simulink model "collection_of_goodies"  (Simulink 5.0)
settings: Solver=ode45  StartTime=0.0  StopTime=10.0  RelTol=1e-3
values from neighbouring files (symbols this model uses):
  c = 4.4*tp/(pi*ts)    [PD_sketch_design.m]
  I = [Ixx,Ixy,Ixz;Iyx,Iyy,Iyz;Izx,Izy,Izz]    [starshotmath.m]
  q0 = [qmatlab(2:4),qmatlab(1)]'    [starshot_DC_KD_setup.m]    (also in starshot_DC_setup.m; temp.m)
  s = tf('s')    [starshot_DC_setup.m]
undefined symbols (not defined in the file or in its folder): a1_T_CMG, a2_T_CMG, a3_T_CMG, AccLim, b1_T_CMG, b2_T_CMG, b3_T_CMG, CFthreshoff, CFthreshon, filt1d, filt1n, filt2d, filt2n, filts1n, filts2d, filts2n, fine, h, h_cos_cmg, h_init, h_sin_cmg, hdmax, hmax, I34, Id, Igm1d, Igm1n, IgmAAFd, invI, invId, Is, Isat, IsatSp, k1_obs, k2_obs, Kt, Kts, lam, Lgm, ls, lt, M34, muE, Ngear, P0, pfd, pfn, q_init, r0, rc_ampl, rc_harm, rc_phase, Rgm, Smin, SmotDrag, spin_init, TachAAFd, TAU_ACS, tr_ampl, tr_harm ... (+8)
libraries: simulink x27, mblibv1 x3, dspinverses x1
(part 1 of 2)
settings Model: LastModifiedBy=E150327

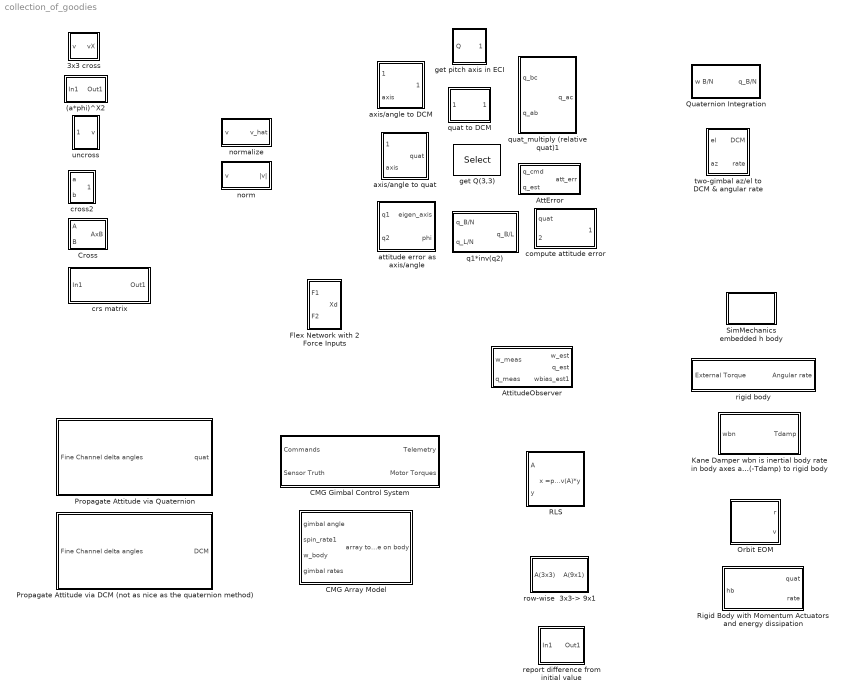
== system collection_of_goodies ==
  " two-gimbal az/el to DCM & angular rate" : Subsystem
  (a*phi)^X2 : Subsystem
      mask Display: disp('3x3 cross')
  3x3 cross : Subsystem
  AttError : Subsystem
  AttitudeObserver : Subsystem
  CMG Array Model : Subsystem
  CMG Gimbal Control System : Subsystem
  Cross : Subsystem
  Flex Network with 2 Force Inputs : Subsystem
  Kane Damper wbn is inertial body rate in body axes apply (-Tdamp) to rigid body : Subsystem
  Orbit EOM : Subsystem
  Propagate Attitude via DCM (not as nice as the quaternion method) : Subsystem
  Propagate Attitude via Quaternion : Subsystem
  Quaternion Integration : Subsystem
  RLS : Subsystem
  Rigid Body with Momentum Actuators and energy dissipation : Subsystem
  SimMechanics embedded h body : Subsystem
  attitude error as axis/angle : Subsystem
  axis/angle to DCM : Subsystem
  axis/angle to quat : Subsystem
  compute attitude error : Subsystem
  cross2 : Subsystem
  crs matrix : Subsystem
  get Q(3,3) : Selector  InputType=Matrix  Elements=9  Rows=3  Columns=3  InputPortWidth=3x3
  get pitch axis in ECI : Subsystem
  norm : Subsystem
  normalize : Subsystem
  q1*inv(q2) : Subsystem
  quat to DCM : Subsystem
      mask Type: Direction Cosine Matrix
      mask Description: Determines the 3x3 Direction Cosine Matrix (DCM) from a 4x1 quaternion orientation vector. The outputted DCM transforms vectors from inertial axes to body axes.  This version corrects the fucked-up MATLAB one.
      mask Help:
      | <p>This block determines the 3x3 Direction Cosine Matrix (DCM) from a 4x1 quaternion orientation vector. The outputted DCM transforms vectors from inertial axes to body axes.  This version corrects the fucked-up MATLAB one</p>
      | 
      | <p>The block input and output contain more than one signal as described below.</p>
      | 
      | <p><H4>Block Vector Input - Quaternion</H4>
      | <ul>
      | <li>q0</li>
      | <li>q1</li>
      | <li>q2</li>
      | <li>q3</li>
      | </ul>
      | </p>
      | 
      | <p><H4>Block Matrix Output - Direction Cosine Matrix  </H4>
      |     <ul>
      |    </ul>
      |    </p>
      mask Display: disp('q to Q')
  quat_multiply (relative quat)1 : Subsystem
  report difference from initial value : Subsystem
  rigid body : Subsystem
  row-wise  3x3-> 9x1 : Subsystem
  uncross : Subsystem

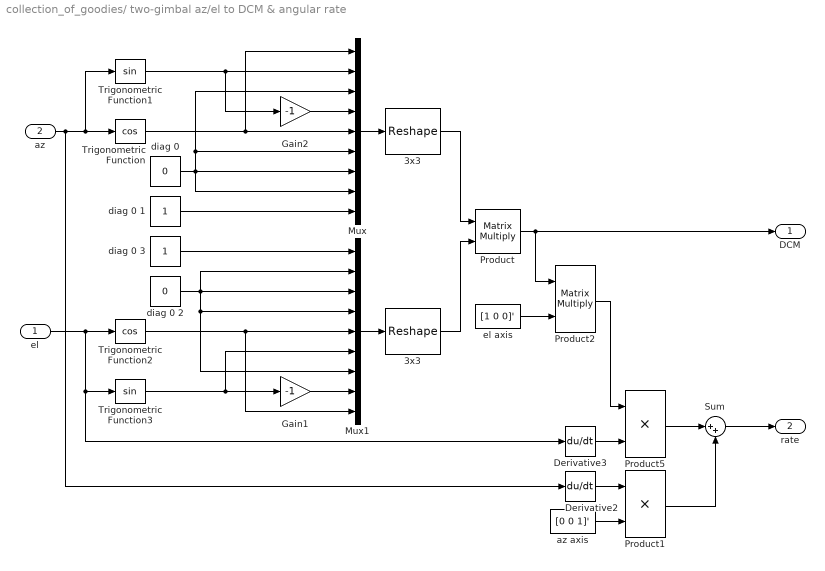
== system collection_of_goodies/ two-gimbal az/el to DCM & angular rate ==
  el : Inport
  az : Inport  Port=2
  3x3 : simulink/Math Operations/Reshape  OutputDimensionality=Customize  OutputDimensions=[3,3]
  "3x3 " : simulink/Math Operations/Reshape  OutputDimensionality=Customize  OutputDimensions=[3,3]
  Derivative2 : Derivative
  Derivative3 : Derivative
  Gain1 : Gain  Gain=-1  SaturateOnIntegerOverflow=on
  Gain2 : Gain  Gain=-1  SaturateOnIntegerOverflow=on
  Mux : Mux  Inputs=9
  Mux1 : Mux  Inputs=9
  Product : Product  Multiplication=Matrix(*)  SaturateOnIntegerOverflow=on
  Product1 : Product  SaturateOnIntegerOverflow=on
  Product2 : Product  Multiplication=Matrix(*)  SaturateOnIntegerOverflow=on
  Product5 : Product  SaturateOnIntegerOverflow=on
  Sum : Sum  Inputs=|++  SaturateOnIntegerOverflow=on
  Trigonometric Function : Trigonometry  Operator=cos
  Trigonometric Function1 : Trigonometry
  Trigonometric Function2 : Trigonometry  Operator=cos
  Trigonometric Function3 : Trigonometry
  az axis : Constant  Value=[0 0 1]'
  "diag 0 " : Constant  Value=0
  diag 0 1 : Constant
  diag 0 2 : Constant  Value=0
  diag 0 3 : Constant
  el axis : Constant  Value=[1 0 0]'
  DCM : Outport
  rate : Outport  Port=2
  wires:
  Mux/1 -> 3x3/1
  3x3/1 -> Product/1
  az/1 -> Trigonometric Function/1, Trigonometric Function1/1, Derivative2/1
  Trigonometric Function/1 -> Mux/1, Mux/5
  Trigonometric Function1/1 -> Gain2/1, Mux/2
  Gain2/1 -> Mux/4
  "diag 0 "/1 -> Mux/8, Mux/7, Mux/6, Mux/3
  diag 0 1/1 -> Mux/9
  Mux1/1 -> "3x3 "/1
  "3x3 "/1 -> Product/2
  el/1 -> Trigonometric Function2/1, Trigonometric Function3/1, Derivative3/1
  diag 0 3/1 -> Mux1/1
  diag 0 2/1 -> Mux1/2, Mux1/3, Mux1/4, Mux1/7
  Trigonometric Function2/1 -> Mux1/5, Mux1/9
  Trigonometric Function3/1 -> Mux1/6, Gain1/1
  Gain1/1 -> Mux1/8
  Product/1 -> DCM/1, Product2/1
  el axis/1 -> Product2/2
  Product2/1 -> Product5/1
  Derivative3/1 -> Product5/2
  Product5/1 -> Sum/1
  Derivative2/1 -> Product1/1
  az axis/1 -> Product1/2
  Product1/1 -> Sum/2
  Sum/1 -> rate/1

== system collection_of_goodies/(a*phi)^X2 ==
  In1 : Inport
  3x3 : simulink/Math Operations/Reshape  OutputDimensionality=Customize  OutputDimensions=[3,3]
  Demux : Demux  Outputs=3
  Gain : Gain  Gain=-1  SaturateOnIntegerOverflow=on
  Gain1 : Gain  Gain=-1  SaturateOnIntegerOverflow=on
  Gain2 : Gain  Gain=-1  SaturateOnIntegerOverflow=on
  Mux : Mux  Inputs=9
  "diag 0 " : Constant  Value=0
  Out1 : Outport
  wires:
  Gain2/1 -> Mux/8
  Demux/1 -> Gain2/1, Mux/6
  Gain1/1 -> Mux/4
  Demux/2 -> Mux/7, Gain/1
  Gain/1 -> Mux/3
  Demux/3 -> Gain1/1, Mux/2
  Mux/1 -> 3x3/1
  "diag 0 "/1 -> Mux/9, Mux/5, Mux/1
  3x3/1 -> Out1/1
  In1/1 -> Demux/1

== system collection_of_goodies/3x3 cross ==
  v : Inport
  Constant1 : Constant  Value=0
  Constant2 : Constant  Value=0
  Constant3 : Constant  Value=0
  Demux : Demux  Outputs=3
  Gain : Gain  Gain=-1  SaturateOnIntegerOverflow=on
  Gain1 : Gain  Gain=-1  SaturateOnIntegerOverflow=on
  Gain2 : Gain  Gain=-1  SaturateOnIntegerOverflow=on
  Matrix Concatenation : simulink/Math Operations/Matrix Concatenation  numInports=3  catMethod=Horizontal
  Mux1 : Mux  Inputs=3
  Mux2 : Mux  Inputs=3
  Mux3 : Mux  Inputs=3
  vX : Outport
  wires:
  v/1 -> Demux/1
  Matrix Concatenation/1 -> vX/1
  Mux3/1 -> Matrix Concatenation/1
  Mux1/1 -> Matrix Concatenation/2
  Mux2/1 -> Matrix Concatenation/3
  Gain/1 -> Mux3/3
  Gain1/1 -> Mux1/1
  Gain2/1 -> Mux2/2
  Constant1/1 -> Mux3/1
  Constant2/1 -> Mux1/2
  Constant3/1 -> Mux2/3
  Demux/3 -> Mux3/2, Gain1/1
  Demux/2 -> Gain/1, Mux2/1
  Demux/1 -> Mux1/3, Gain2/1

== system collection_of_goodies/AttError ==
  q_cmd : Inport  PortDimensions=4
  q_est : Inport  Port=2  PortDimensions=4
  Demux : Demux
  Gain : Gain  Gain=2  SaturateOnIntegerOverflow=on
  Mux : Mux  Inputs=3
  Terminator : Terminator
  qconjMult : Subsystem
  att_err : Outport
  wires:
  q_cmd/1 -> qconjMult/1(q_cmd)
  q_est/1 -> qconjMult/2(q_est)
  qconjMult/1(q_err) -> Demux/1
  Demux/1 -> Mux/1
  Demux/2 -> Mux/2
  Demux/3 -> Mux/3
  Mux/1 -> Gain/1
  Gain/1 -> att_err/1
  Demux/4 -> Terminator/1

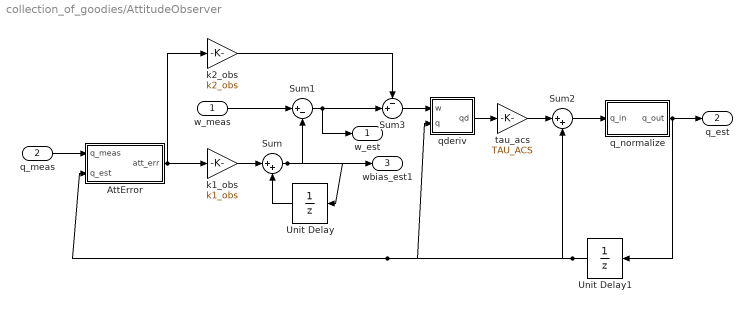
== system collection_of_goodies/AttitudeObserver ==
  w_meas : Inport  PortDimensions=3
  q_meas : Inport  Port=2  PortDimensions=4
  AttError : Subsystem
  Sum : Sum  Inputs=|++  SaturateOnIntegerOverflow=on  InputSameDT=on
  Sum1 : Sum  Inputs=|+-  SaturateOnIntegerOverflow=on  InputSameDT=on
  Sum2 : Sum  Inputs=|++  SaturateOnIntegerOverflow=on  InputSameDT=on
  Sum3 : Sum  Inputs=-+|  SaturateOnIntegerOverflow=on  InputSameDT=on
  Unit Delay : UnitDelay  Orientation=left  X0=[0;0;0]  SampleTime=TAU_ACS
  Unit Delay1 : UnitDelay  Orientation=left  X0=q0  SampleTime=TAU_ACS
  k1_obs : Gain  Gain=k1_obs  SaturateOnIntegerOverflow=on
  k2_obs : Gain  Gain=k2_obs  SaturateOnIntegerOverflow=on
  q_normalize : Subsystem
  qderiv : Subsystem
  tau_acs : Gain  Gain=TAU_ACS  SaturateOnIntegerOverflow=on
  w_est : Outport
  q_est : Outport  Port=2
  wbias_est1 : Outport  Port=3
  wires:
  q_meas/1 -> AttError/1(q_meas)
  k1_obs/1 -> Sum/1
  Unit Delay/1 -> Sum/2
  AttError/1(att_err) -> k1_obs/1, k2_obs/1
  Sum/1 -> Unit Delay/1, Sum1/2, wbias_est1/1
  w_meas/1 -> Sum1/1
  qderiv/1(qd) -> tau_acs/1
  tau_acs/1 -> Sum2/1
  Sum2/1 -> q_normalize/1(q_in)
  k2_obs/1 -> Sum3/1
  Sum3/1 -> qderiv/1(w)
  Unit Delay1/1 -> AttError/2(q_est), qderiv/2(q), Sum2/2
  Sum1/1 -> Sum3/2, w_est/1
  q_normalize/1(q_out) -> Unit Delay1/1, q_est/1

== system collection_of_goodies/CMG Array Model ==
  note: this value times the inverse fo the spacecraft
      | inertia matrix is added to the body rate (w_body)
      | derivative.
  gimbal angle : Inport  PortDimensions=6
  spin_rate1 : Inport  Port=2  PortDimensions=6
  w_body : Inport  Port=3  PortDimensions=6
  gimbal rates : Inport  Port=4  PortDimensions=6
  Array_Steering : Subsystem
  ComputeCMGMomentum : Subsystem
  Sum : Sum  Inputs=++|  SaturateOnIntegerOverflow=on  InputSameDT=on
  WxH (gyroscopic torque) : Subsystem
  array torque on body : Outport
  wires:
  gimbal angle/1 -> Array_Steering/3(gim_ang_meas), ComputeCMGMomentum/2(gim_ang_meas)
  spin_rate1/1 -> Array_Steering/2(spin_rate_meas), ComputeCMGMomentum/1(spin_rate_meas)
  ComputeCMGMomentum/1(H_cmg) -> WxH (gyroscopic torque)/2(v2)
  w_body/1 -> WxH (gyroscopic torque)/1(v1)
  Sum/1 -> array torque on body/1
  WxH (gyroscopic torque)/1(v1xv2) -> Sum/2
  Array_Steering/1(torque) -> Sum/1
  gimbal rates/1 -> Array_Steering/1(gimbal_rate)

== system collection_of_goodies/CMG Gimbal Control System ==
  Commands : Inport
  Sensor Truth : Inport  Orientation=left  Port=2
  Actuator : Subsystem
  Control : Subsystem
  Drive : Subsystem
  Sensor : Subsystem  Orientation=left
  Telemetry : Outport  InitialOutput=0
  Motor Torques : Outport  Port=2  InitialOutput=0
  wires:
  Actuator/1(Current) -> Drive/1(Current)
  Control/1(CurrentCmd) -> Drive/2(CurrentCmd)
  Drive/1(Vcoil) -> Actuator/1(Vcoil)
  Actuator/2(Torque) -> Motor Torques/1
  Drive/2(CurSense) -> Sensor/2(CurSense)
  Control/2(TachComm) -> Sensor/1(TachComm)
  Sensor/1(Sensor) -> Control/2(Feedback)
  Commands/1 -> Control/1(Command)
  Sensor Truth/1 -> Sensor/3(Truth), Actuator/2(Truth), Telemetry/1

== system collection_of_goodies/Cross ==
  A : Inport
  B : Inport  Port=2
  Mux4 : Mux  Inputs=3
  Product{,1..5} (6 alike) : Product  SaturateOnIntegerOverflow=on  InputSameDT=on
  Sum : Sum  Inputs=+-  SaturateOnIntegerOverflow=on  InputSameDT=on
  Sum1 : Sum  Inputs=+-  SaturateOnIntegerOverflow=on  InputSameDT=on
  Sum2 : Sum  Inputs=+-  SaturateOnIntegerOverflow=on  InputSameDT=on
  demux2 : Demux  Outputs=3
  demux3 : Demux  Outputs=3
  AxB : Outport  InitialOutput=0
  wires:
  Mux4/1 -> AxB/1
  Sum2/1 -> Mux4/3
  Sum1/1 -> Mux4/2
  Sum/1 -> Mux4/1
  Product5/1 -> Sum2/2
  Product4/1 -> Sum2/1
  Product3/1 -> Sum1/2
  Product2/1 -> Sum1/1
  Product1/1 -> Sum/2
  Product/1 -> Sum/1
  demux3/1 -> Product5/2, Product2/2
  demux2/2 -> Product5/1, Product/1
  demux3/2 -> Product4/2, Product1/2
  demux2/1 -> Product4/1, Product3/1
  demux3/3 -> Product3/2, Product/2
  demux2/3 -> Product2/1, Product1/1
  B/1 -> demux3/1
  A/1 -> demux2/1

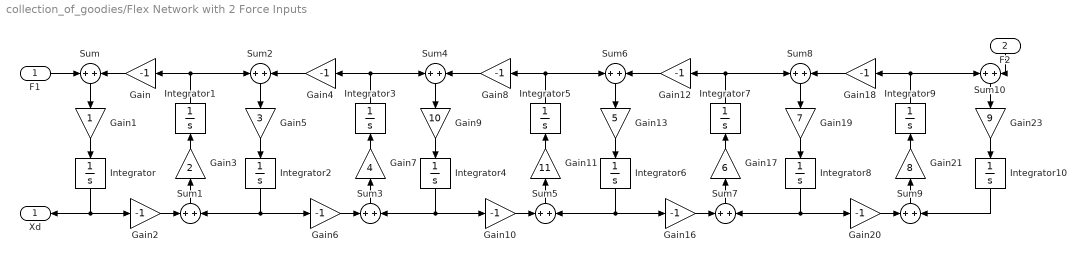
== system collection_of_goodies/Flex Network with 2 Force Inputs ==
  F1 : Inport
  F2 : Inport  Orientation=down  Port=2
  Gain{,4,8,12,18} (5 alike) : Gain  Orientation=left  Gain=-1  SaturateOnIntegerOverflow=on
  Gain1 : Gain  Orientation=down  SaturateOnIntegerOverflow=on
  Gain{2,6,10,16,20} (5 alike) : Gain  Gain=-1  SaturateOnIntegerOverflow=on
  Gain11 : Gain  Orientation=up  Gain=11  SaturateOnIntegerOverflow=on
  Gain13 : Gain  Orientation=down  Gain=5  SaturateOnIntegerOverflow=on
  Gain17 : Gain  Orientation=up  Gain=6  SaturateOnIntegerOverflow=on
  Gain19 : Gain  Orientation=down  Gain=7  SaturateOnIntegerOverflow=on
  Gain21 : Gain  Orientation=up  Gain=8  SaturateOnIntegerOverflow=on
  Gain23 : Gain  Orientation=down  Gain=9  SaturateOnIntegerOverflow=on
  Gain3 : Gain  Orientation=up  Gain=2  SaturateOnIntegerOverflow=on
  Gain5 : Gain  Orientation=down  Gain=3  SaturateOnIntegerOverflow=on
  Gain7 : Gain  Orientation=up  Gain=4  SaturateOnIntegerOverflow=on
  Gain9 : Gain  Orientation=down  Gain=10  SaturateOnIntegerOverflow=on
  Integrator{,2,4,6,8,10} (6 alike) : Integrator  Orientation=down
  Integrator{1,3,5,7,9} (5 alike) : Integrator  Orientation=up
  Sum{,2,4,6,8,10} (6 alike) : Sum  Orientation=down  Inputs=+|+  SaturateOnIntegerOverflow=on  InputSameDT=on
  Sum{1,3,5,7,9} (5 alike) : Sum  Orientation=up  Inputs=+|+  SaturateOnIntegerOverflow=on  InputSameDT=on
  Xd : Outport  Orientation=left
  wires:
  F1/1 -> Sum/1
  Gain/1 -> Sum/2
  Sum/1 -> Gain1/1
  Gain1/1 -> Integrator/1
  Gain2/1 -> Sum1/1
  Integrator/1 -> Xd/1, Gain2/1
  Sum1/1 -> Gain3/1
  Gain3/1 -> Integrator1/1
  Integrator1/1 -> Gain/1, Sum2/1
  Gain4/1 -> Sum2/2
  Sum2/1 -> Gain5/1
  Gain5/1 -> Integrator2/1
  Gain6/1 -> Sum3/1
  Integrator2/1 -> Gain6/1, Sum1/2
  Sum3/1 -> Gain7/1
  Gain7/1 -> Integrator3/1
  Integrator3/1 -> Gain4/1, Sum4/1
  Gain8/1 -> Sum4/2
  Sum4/1 -> Gain9/1
  Gain9/1 -> Integrator4/1
  Gain10/1 -> Sum5/1
  Integrator4/1 -> Gain10/1, Sum3/2
  Sum5/1 -> Gain11/1
  Gain11/1 -> Integrator5/1
  Integrator5/1 -> Gain8/1, Sum6/1
  Gain12/1 -> Sum6/2
  Sum6/1 -> Gain13/1
  Gain13/1 -> Integrator6/1
  Gain16/1 -> Sum7/1
  Integrator6/1 -> Gain16/1, Sum5/2
  Sum7/1 -> Gain17/1
  Gain17/1 -> Integrator7/1
  Integrator7/1 -> Gain12/1, Sum8/1
  Gain18/1 -> Sum8/2
  Sum8/1 -> Gain19/1
  Gain19/1 -> Integrator8/1
  Gain20/1 -> Sum9/1
  Integrator8/1 -> Gain20/1, Sum7/2
  Sum9/1 -> Gain21/1
  Gain21/1 -> Integrator9/1
  Integrator9/1 -> Gain18/1, Sum10/1
  Sum10/1 -> Gain23/1
  Gain23/1 -> Integrator10/1
  Integrator10/1 -> Sum9/2
  F2/1 -> Sum10/2

== system collection_of_goodies/Kane Damper wbn is inertial body rate in body axes apply (-Tdamp) to rigid body ==
  wbn : Inport
  Big-dog Kane damping : Gain  Gain=c  SaturateOnIntegerOverflow=on
  Cross1 : Subsystem  Orientation=left
  Id : Gain  Orientation=left  Gain=Id  Multiplication=Matrix(K*u)  SaturateOnIntegerOverflow=on
  Id inverse : Gain  Gain=inv(Id)  Multiplication=Matrix(K*u)  SaturateOnIntegerOverflow=on
  Sum8 : Sum  Inputs=|+-  SaturateOnIntegerOverflow=on  InputSameDT=on
  Sum9 : Sum  Inputs=|+-  SaturateOnIntegerOverflow=on  InputSameDT=on
  "wdmp dot -> wdmp" : Integrator  InitialCondition=wd_init
  Tdamp : Outport
  wires:
  wbn/1 -> Cross1/1(A), Sum9/1
  Id inverse/1 -> "wdmp dot -> wdmp"/1
  "wdmp dot -> wdmp"/1 -> Sum9/2, Id/1
  Id/1 -> Cross1/2(B)
  Cross1/1(AxB) -> Sum8/2
  Sum8/1 -> Id inverse/1
  Sum9/1 -> Big-dog Kane damping/1
  Big-dog Kane damping/1 -> Tdamp/1, Sum8/1

== system collection_of_goodies/Orbit EOM ==
  Demux : Demux  Outputs=3
  Earth's grav constant : Constant  Value=muE
  Gain : Gain  Gain=-1  SaturateOnIntegerOverflow=on
  Integrator : Integrator  InitialCondition=v0
  Integrator1 : Integrator  InitialCondition=r0
  Product : Product  Inputs=*/  SaturateOnIntegerOverflow=on
  Product1 : Product  Inputs=***  SaturateOnIntegerOverflow=on
  Product2 : Product  Inputs=**  SaturateOnIntegerOverflow=on
  Scope : Scope  NumInputPorts=3
      settings: YMin=-5~-5~-5  YMax=5~5~5
  norm : Subsystem  Orientation=left
  r : Outport
  v : Outport  Port=2
  wires:
  norm/1(|v|) -> Product1/3, Product1/2, Product1/1
  Demux/3 -> Scope/3
  Demux/2 -> Scope/2
  Demux/1 -> Scope/1
  Gain/1 -> Product2/1
  Integrator/1 -> v/1, Integrator1/1
  Product2/1 -> Integrator/1
  Product/1 -> Gain/1
  Integrator1/1 -> r/1, Demux/1, norm/1(v), Product2/2
  Product1/1 -> Product/2
  Earth's grav constant/1 -> Product/1

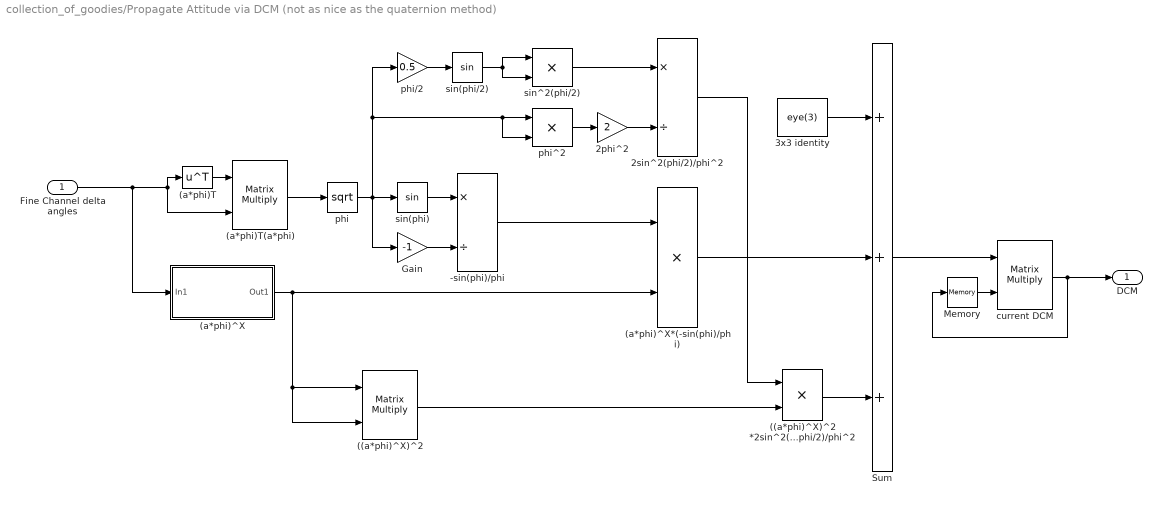
== system collection_of_goodies/Propagate Attitude via DCM (not as nice as the quaternion method) ==
  Fine Channel delta angles : Inport
  ((a*phi)^X)^2 : Product  Multiplication=Matrix(*)  SaturateOnIntegerOverflow=on  InputSameDT=on
  "((a*phi)^X)^2 *2sin^2(phi/2)/phi^2 " : Product  SaturateOnIntegerOverflow=on  InputSameDT=on
  (a*phi)T : Math  Operator=transpose
  (a*phi)T(a*phi) : Product  Multiplication=Matrix(*)  SaturateOnIntegerOverflow=on  InputSameDT=on
  (a*phi)^X : Subsystem
      mask Display: disp('3x3 cross matrix')
  (a*phi)^X*(-sin(phi)/phi) : Product  SaturateOnIntegerOverflow=on  InputSameDT=on
  -sin(phi)/phi : Product  Inputs=*/  SaturateOnIntegerOverflow=on  InputSameDT=on
  2phi^2 : Gain  Gain=2  SaturateOnIntegerOverflow=on
  2sin^2(phi/2)/phi^2 : Product  Inputs=*/  SaturateOnIntegerOverflow=on  InputSameDT=on
  3x3 identity : Constant  Value=eye(3)
  Gain : Gain  Gain=-1  SaturateOnIntegerOverflow=on
  Memory : Memory  X0=eye(3)
  Sum : Sum  Inputs=+++  SaturateOnIntegerOverflow=on  InputSameDT=on
  current DCM : Product  Multiplication=Matrix(*)  SaturateOnIntegerOverflow=on  InputSameDT=on
  phi : Math  Operator=sqrt
  phi/2 : Gain  Gain=0.5  SaturateOnIntegerOverflow=on
  phi^2 : Product  SaturateOnIntegerOverflow=on  InputSameDT=on
  sin(phi) : Trigonometry
  sin(phi/2) : Trigonometry
  sin^2(phi/2) : Product  SaturateOnIntegerOverflow=on  InputSameDT=on
  DCM : Outport
  wires:
  Fine Channel delta angles/1 -> (a*phi)T(a*phi)/2, (a*phi)T/1, (a*phi)^X/1(In1)
  (a*phi)T/1 -> (a*phi)T(a*phi)/1
  (a*phi)T(a*phi)/1 -> phi/1
  (a*phi)^X/1(Out1) -> (a*phi)^X*(-sin(phi)/phi)/2, ((a*phi)^X)^2/1, ((a*phi)^X)^2/2
  3x3 identity/1 -> Sum/1
  phi/1 -> Gain/1, sin(phi)/1, phi/2/1, phi^2/1, phi^2/2
  sin(phi)/1 -> -sin(phi)/phi/1
  Gain/1 -> -sin(phi)/phi/2
  -sin(phi)/phi/1 -> (a*phi)^X*(-sin(phi)/phi)/1
  (a*phi)^X*(-sin(phi)/phi)/1 -> Sum/2
  phi/2/1 -> sin(phi/2)/1
  sin(phi/2)/1 -> sin^2(phi/2)/1, sin^2(phi/2)/2
  phi^2/1 -> 2phi^2/1
  2phi^2/1 -> 2sin^2(phi/2)/phi^2/2
  sin^2(phi/2)/1 -> 2sin^2(phi/2)/phi^2/1
  2sin^2(phi/2)/phi^2/1 -> "((a*phi)^X)^2 *2sin^2(phi/2)/phi^2 "/1
  ((a*phi)^X)^2/1 -> "((a*phi)^X)^2 *2sin^2(phi/2)/phi^2 "/2
  Memory/1 -> current DCM/2
  current DCM/1 -> Memory/1, DCM/1
  Sum/1 -> current DCM/1
  "((a*phi)^X)^2 *2sin^2(phi/2)/phi^2 "/1 -> Sum/3

== system collection_of_goodies/Propagate Attitude via Quaternion ==
  Fine Channel delta angles : Inport
  (a*phi)T : Math  Operator=transpose
  (a*phi)T(a*phi) : Product  Multiplication=Matrix(*)  SaturateOnIntegerOverflow=on  InputSameDT=on
  Constant : Constant
  Demux : Demux  Outputs=3
  Gain : Gain  Gain=0.5  SaturateOnIntegerOverflow=on
  Mux : Mux
  Sum : Sum  Inputs=|-+  SaturateOnIntegerOverflow=on  InputSameDT=on
  previous value : Memory  X0=[0 0 0 1]'
  q_normalize : Subsystem
  quat_multiply : Subsystem
  quat : Outport
  wires:
  (a*phi)T/1 -> (a*phi)T(a*phi)/1
  previous value/1 -> quat_multiply/2(q_ab)
  quat_multiply/1(q_ac) -> q_normalize/1(q_in)
  q_normalize/1(q_out) -> previous value/1, quat/1
  Sum/1 -> Mux/4
  Fine Channel delta angles/1 -> Gain/1
  Constant/1 -> Sum/2
  (a*phi)T(a*phi)/1 -> Sum/1
  Gain/1 -> (a*phi)T/1, (a*phi)T(a*phi)/2, Demux/1
  Demux/1 -> Mux/1
  Demux/2 -> Mux/2
  Demux/3 -> Mux/3
  Mux/1 -> quat_multiply/1(q_bc)

== system collection_of_goodies/Quaternion Integration ==
  w B/N : Inport
  Integrator1 : Integrator  InitialCondition=q0
  q_normalize : Subsystem
  qderiv : Subsystem
  q_B/N : Outport
  wires:
  qderiv/1(qd) -> Integrator1/1
  Integrator1/1 -> q_normalize/1(q_in)
  q_normalize/1(q_out) -> q_B/N/1, qderiv/2(q)
  w B/N/1 -> qderiv/1(w)

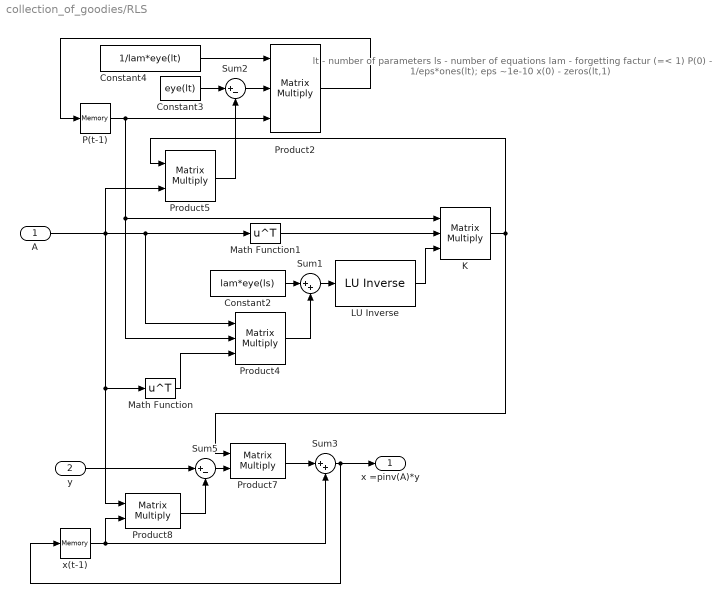
== system collection_of_goodies/RLS ==
  note: lt - number of parameters
      | ls - number of equations
      | lam - forgetting factur (=< 1)
      | P(0) - 1/eps*ones(lt); eps ~1e-10
      | x(0) - zeros(lt,1)
  A : Inport
  y : Inport  Port=2
  " LU Inverse" : dspinverses/ LU Inverse
  Constant2 : Constant  Value=lam*eye(ls)
  Constant3 : Constant  Value=eye(lt)
  Constant4 : Constant  Value=1/lam*eye(lt)
  K : Product  Inputs=3  Multiplication=Matrix(*)  SaturateOnIntegerOverflow=on
  Math Function : Math  Operator=transpose
  Math Function1 : Math  Operator=transpose
  P(t-1) : Memory  X0=P0  InheritSampleTime=on
  Product2 : Product  Inputs=3  Multiplication=Matrix(*)  SaturateOnIntegerOverflow=on
  Product4 : Product  Inputs=3  Multiplication=Matrix(*)  SaturateOnIntegerOverflow=on
  Product5 : Product  Multiplication=Matrix(*)  SaturateOnIntegerOverflow=on
  Product7 : Product  Multiplication=Matrix(*)  SaturateOnIntegerOverflow=on
  Product8 : Product  Multiplication=Matrix(*)  SaturateOnIntegerOverflow=on
  Sum1 : Sum  Inputs=|++  SaturateOnIntegerOverflow=on
  Sum2 : Sum  Inputs=|+-  SaturateOnIntegerOverflow=on
  Sum3 : Sum  Inputs=|++  SaturateOnIntegerOverflow=on
  Sum5 : Sum  Inputs=|+-  SaturateOnIntegerOverflow=on
  x(t-1) : Memory  X0=x0  InheritSampleTime=on
  x =pinv(A)*y : Outport
  wires:
  A/1 -> Product8/1, Math Function/1, Product5/2, Math Function1/1, Product4/1
  P(t-1)/1 -> K/1, Product4/2, Product2/3
  " LU Inverse"/1 -> K/3
  Constant2/1 -> Sum1/1
  Product4/1 -> Sum1/2
  Math Function/1 -> Product4/3
  Sum1/1 -> " LU Inverse"/1
  Constant4/1 -> Product2/1
  Sum2/1 -> Product2/2
  Constant3/1 -> Sum2/1
  K/1 -> Product7/1, Product5/1
  Product5/1 -> Sum2/2
  Product2/1 -> P(t-1)/1
  x(t-1)/1 -> Sum3/2, Product8/2
  Sum3/1 -> x(t-1)/1, x =pinv(A)*y/1
  Product7/1 -> Sum3/1
  Sum5/1 -> Product7/2
  Product8/1 -> Sum5/2
  Math Function1/1 -> K/2
  y/1 -> Sum5/1

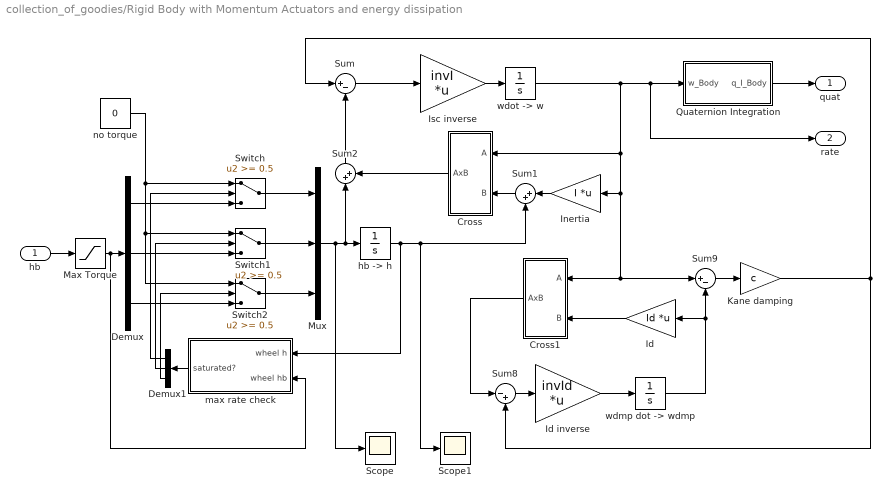
== system collection_of_goodies/Rigid Body with Momentum Actuators and energy dissipation ==
  hb : Inport
  Cross : Subsystem  Orientation=left
  Cross1 : Subsystem  Orientation=left
  Demux : Demux  Outputs=3
  Demux1 : Demux  Orientation=left  Outputs=3
  Id : Gain  Orientation=left  Gain=Id  Multiplication=Matrix(K*u)  SaturateOnIntegerOverflow=on
  Id inverse : Gain  Gain=invId  Multiplication=Matrix(K*u)  SaturateOnIntegerOverflow=on
  Inertia : Gain  Orientation=left  Gain=I  Multiplication=Matrix(K*u)  SaturateOnIntegerOverflow=on
  Isc inverse : Gain  Gain=invI  Multiplication=Matrix(K*u)  SaturateOnIntegerOverflow=on
  Kane damping : Gain  Gain=c  SaturateOnIntegerOverflow=on
  Max Torque : Saturate  UpperLimit=hdmax  LowerLimit=-hdmax
  Mux : Mux  Inputs=3
  Quaternion Integration : Subsystem
  Scope : Scope
      settings: YMin=-0.01  YMax=0.03  SaveName=ScopeData2
  Scope1 : Scope
      settings: YMin=-0.01  YMax=0.03  SaveName=ScopeData3
  Sum : Sum  Inputs=|+-  SaturateOnIntegerOverflow=on  InputSameDT=on
  Sum1 : Sum  Orientation=left  Inputs=|++  SaturateOnIntegerOverflow=on  InputSameDT=on
  Sum2 : Sum  Orientation=up  Inputs=|++  SaturateOnIntegerOverflow=on  InputSameDT=on
  Sum8 : Sum  Inputs=|-+  SaturateOnIntegerOverflow=on  InputSameDT=on
  Sum9 : Sum  Inputs=|+-  SaturateOnIntegerOverflow=on  InputSameDT=on
  Switch : Switch  Threshold=0.5  SaturateOnIntegerOverflow=on  InputSameDT=on
  Switch1 : Switch  Threshold=0.5  SaturateOnIntegerOverflow=on  InputSameDT=on
  Switch2 : Switch  Threshold=0.5  SaturateOnIntegerOverflow=on  InputSameDT=on
  "hb -> h" : Integrator  InitialCondition=h_init
  max rate check : Subsystem  Orientation=left
  no torque : Constant  Value=0
  "wdmp dot -> wdmp" : Integrator  InitialCondition=wdn_init
  "wdot -> w" : Integrator  InitialCondition=wbn_init
  quat : Outport
  rate : Outport  Port=2
  wires:
  Sum/1 -> Isc inverse/1
  "wdot -> w"/1 -> Cross/1(A), Inertia/1, Cross1/1(A), Sum9/1, Quaternion Integration/1(w_Body), rate/1
  Inertia/1 -> Sum1/1
  Sum1/1 -> Cross/2(B)
  "hb -> h"/1 -> max rate check/1(wheel h), Sum1/2, Scope1/1
  Id inverse/1 -> "wdmp dot -> wdmp"/1
  "wdmp dot -> wdmp"/1 -> Sum9/2, Id/1
  Id/1 -> Cross1/2(B)
  Sum8/1 -> Id inverse/1
  Sum9/1 -> Kane damping/1
  Isc inverse/1 -> "wdot -> w"/1
  Sum2/1 -> Sum/2
  Cross/1(AxB) -> Sum2/2
  Cross1/1(AxB) -> Sum8/1
  hb/1 -> Max Torque/1
  Kane damping/1 -> Sum8/2, Sum/1
  Quaternion Integration/1(q_I_Body) -> quat/1
  Mux/1 -> "hb -> h"/1, Sum2/1, Scope/1
  Max Torque/1 -> Demux/1, max rate check/2(wheel hb)
  max rate check/1(saturated?) -> Demux1/1
  Demux1/1 -> Switch/2
  Demux1/2 -> Switch1/2
  Demux1/3 -> Switch2/2
  no torque/1 -> Switch/1, Switch1/1, Switch2/1
  Demux/1 -> Switch/3
  Demux/2 -> Switch1/3
  Demux/3 -> Switch2/3
  Switch/1 -> Mux/1
  Switch1/1 -> Mux/2
  Switch2/1 -> Mux/3

== system collection_of_goodies/SimMechanics embedded h body ==
  Body : mblibv1/Bodies/Body  PhysicalDomain=mechanical  SubClassName=Unknown  PortType=workingframe  LConnTagsString=CS1|CS4  RConnTagsString=CS2|CS3  DialogClass=MechanicalBodyBlock  Mass=M34  MassUnits=kg  InertiaUnits=kg*m^2  Inertia=I34  Shape=Cylinder  ShapeDims=[1 1]  ShapeUnits=m  ShapeUse=false  Density=1  DensityUnits=kg/m^3  DensityUse=false  CG=Left$CG$R34$WORLD$WORLD$m$[0 0 0]$Euler X-Y-Z$deg$WORLD$false  WorkingFrames=Left$CS1$[0 -1 0]$CG$CG$m$[0 0 0]$Euler X-Y-Z$deg$WORLD$true#Right$CS2$[1 0 0]$CG$CG$m$[0 0 0]$Euler X-Y-Z$deg$WORLD$true#Right$CS3$[-1 0 0]$CG$CG$m$[0 0 0]$Euler X-Y-Z$deg$WORLD$true#Left$CS4$[0 1 0]$CG$CG$m$[0 0 0]$Euler X-Y-Z$deg$WORLD$true
  Body Actuator : mblibv1/Sensors &  Actuators/Body Actuator  Tag=__orphan__  PortType=blob  PhysicalDomain=Mechanical  ActuationStyle=Force  AngleUnits=deg  ArcVelocityUnits=deg/s  ArcAccelerationUnits=deg/s^2  CoordPositionUnits=m  VelocityUnits=m/s  AccelerationUnits=m/s^2  ForceUnits=N  TorqueUnits=N-m  DialogClass=MechanicalActuatorBlock  ReferenceFrame=Local (Body CS)  Angle=off  CoordPosition=on  Force=off  Torque=on
  Body Sensor : mblibv1/Sensors &  Actuators/Body Sensor  Tag=__orphan__  PortType=blob  PhysicalDomain=Mechanical  Muxed=on  Pose=off  Angle=on  AngleUnits=deg  ArcVelocity=on  ArcVelocityUnits=rad/s  ArcAcceleration=off  ArcAccelerationUnits=deg/s^2  CoordPosition=off  CoordPositionUnits=m  Velocity=off  VelocityUnits=m/s  Acceleration=off  AccelerationUnits=m/s^2  Quaternion=on  QuaternionDT=off  QuaternionDDT=off  QuaternionUnits=off  OutputVector=[ 3 ]  DialogClass=MechanicalSensorBlock  ReferenceFrame=Local (Body CS)
  Gain : Gain  Orientation=left  Gain=-1  SaturateOnIntegerOverflow=on
  cross2 : Subsystem
  embedded momentum : Constant  Value=h
  CS1 : PMIOPort  Port=1  Side=left
  CS2 : PMIOPort  Orientation=left  Port=2  Side=right
  wires:
  Body Sensor/1 -> cross2/1(a)
  embedded momentum/1 -> cross2/2(b)
  cross2/1(a x b) -> Gain/1
  Gain/1 -> Body Actuator/1
  connections:
  Body Actuator/RConn1 -- Body/LConn2
  Body/RConn2 -- Body Sensor/LConn1
  CS1/RConn1 -- Body/LConn1
  CS2/RConn1 -- Body/RConn1

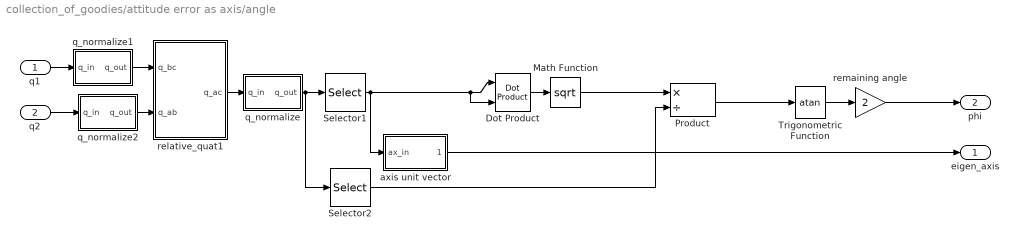
== system collection_of_goodies/attitude error as axis/angle ==
  q1 : Inport
  q2 : Inport  Port=2
  Dot Product : simulink/Math Operations/Dot Product
  Math Function : Math  Operator=sqrt
  Product : Product  Inputs=*/  SaturateOnIntegerOverflow=on
  Selector1 : Selector  Elements=[1 2 3]  InputPortWidth=4
  Selector2 : Selector  Elements=[4]  InputPortWidth=4
  Trigonometric Function : Trigonometry  Operator=atan
  axis unit vector : Subsystem  TreatAsAtomicUnit=on
  q_normalize : Subsystem  TreatAsAtomicUnit=on
  q_normalize1 : Subsystem  TreatAsAtomicUnit=on
  q_normalize2 : Subsystem  TreatAsAtomicUnit=on
  relative_quat1 : Subsystem  TreatAsAtomicUnit=on
  remaining angle : Gain  Gain=2  SaturateOnIntegerOverflow=on
  eigen_axis : Outport
  phi : Outport  Port=2
  wires:
  q1/1 -> q_normalize1/1(q_in)
  relative_quat1/1(q_ac) -> q_normalize/1(q_in)
  q_normalize/1(q_out) -> Selector1/1, Selector2/1
  axis unit vector/1(ax_out) -> eigen_axis/1
  Dot Product/1 -> Math Function/1
  q_normalize1/1(q_out) -> relative_quat1/1(q_bc)
  q_normalize2/1(q_out) -> relative_quat1/2(q_ab)
  Selector1/1 -> axis unit vector/1(ax_in), Dot Product/1, Dot Product/2
  Trigonometric Function/1 -> remaining angle/1
  remaining angle/1 -> phi/1
  q2/1 -> q_normalize2/1(q_in)
  Math Function/1 -> Product/1
  Selector2/1 -> Product/2
  Product/1 -> Trigonometric Function/1

== system collection_of_goodies/axis/angle to DCM ==
  angle : Inport
  axis : Inport  Port=2
  Constant : Constant
  Math Function : Math  Operator=transpose
  Sum : Sum  Inputs=+-|  SaturateOnIntegerOverflow=on
  Sum1 : Sum  Inputs=+++  SaturateOnIntegerOverflow=on
  Trigonometric Function : Trigonometry  Operator=cos
  Trigonometric Function1 : Trigonometry
  crs matrix : Subsystem
  crs matrix1 : Subsystem
  g*g' : Product  Multiplication=Matrix(*)  SaturateOnIntegerOverflow=on
  g*g'1 : Product  SaturateOnIntegerOverflow=on
  g*g'2 : Product  SaturateOnIntegerOverflow=on
  dircos : Outport
  wires:
  angle/1 -> Trigonometric Function/1, Trigonometric Function1/1
  Trigonometric Function/1 -> Sum/2, crs matrix1/1(make)
  Constant/1 -> Sum/1
  Sum/1 -> g*g'1/2
  axis/1 -> g*g'/1, Math Function/1, crs matrix/1(In1)
  Math Function/1 -> g*g'/2
  g*g'/1 -> g*g'1/1
  g*g'1/1 -> Sum1/2
  Trigonometric Function1/1 -> g*g'2/2
  crs matrix/1(Out1) -> g*g'2/1
  Sum1/1 -> dircos/1
  crs matrix1/1(3x3) -> Sum1/1
  g*g'2/1 -> Sum1/3

== system collection_of_goodies/axis/angle to quat ==
  angle : Inport
  axis : Inport  Port=2
  Gain : Gain  Gain=0.5  SaturateOnIntegerOverflow=on
  Mux : Mux  Inputs=2
  Product : Product  SaturateOnIntegerOverflow=on
  Trigonometric Function : Trigonometry
  Trigonometric Function1 : Trigonometry  Operator=cos
  quat : Outport
  wires:
  Mux/1 -> quat/1
  Trigonometric Function1/1 -> Mux/2
  Product/1 -> Mux/1
  Trigonometric Function/1 -> Product/2
  axis/1 -> Product/1
  Gain/1 -> Trigonometric Function1/1, Trigonometric Function/1
  angle/1 -> Gain/1

== system collection_of_goodies/compute attitude error ==
  quat : Inport
  quat_cmd : Inport  Port=2
  Demux : Demux
  Mux : Mux  Inputs=3
  Mux1 : Mux  Inputs=2
  quat_multiply (relative quat) : Subsystem
  reverse : Gain  Gain=-1  SaturateOnIntegerOverflow=on
  quat error : Outport
  wires:
  quat/1 -> quat_multiply (relative quat)/1(q_bc)
  quat_cmd/1 -> Demux/1
  Demux/1 -> Mux/1
  Demux/2 -> Mux/2
  Demux/3 -> Mux/3
  Demux/4 -> reverse/1
  Mux/1 -> Mux1/1
  Mux1/1 -> quat_multiply (relative quat)/2(q_ab)
  reverse/1 -> Mux1/2
  quat_multiply (relative quat)/1(q_ac) -> quat error/1

== system collection_of_goodies/cross2 ==
  a : Inport
  b : Inport  Port=2
  Demux : Demux  Outputs=3
  Demux1 : Demux  Outputs=3
  Fcn : Fcn  Expr=-u(3)*u(5)+u(2)*u(6)
  Fcn1 : Fcn  Expr=u(3)*u(4)-u(1)*u(6)
  Fcn2 : Fcn  Expr=-u(2)*u(4)+u(1)*u(5)
  Mux : Mux  Inputs=6
  Mux1 : Mux  Inputs=3
  a x b : Outport
  wires:
  Mux/1 -> Fcn/1, Fcn1/1, Fcn2/1
  Mux1/1 -> a x b/1
  Fcn/1 -> Mux1/1
  Fcn1/1 -> Mux1/2
  Fcn2/1 -> Mux1/3
  Demux/1 -> Mux/1
  Demux/2 -> Mux/2
  Demux/3 -> Mux/3
  a/1 -> Demux/1
  Demux1/1 -> Mux/4
  Demux1/2 -> Mux/5
  Demux1/3 -> Mux/6
  b/1 -> Demux1/1

== system collection_of_goodies/crs matrix ==
  In1 : Inport
  Constant : Constant  Value=0
  Demux : Demux  Outputs=3
  Gain : Gain  Gain=-1  SaturateOnIntegerOverflow=on
  Gain1 : Gain  Gain=-1  SaturateOnIntegerOverflow=on
  Gain2 : Gain  Gain=-1  SaturateOnIntegerOverflow=on
  Matrix Concatenation : simulink/Math Operations/Matrix Concatenation  numInports=3  catMethod=Horizontal
  Mux : Mux  Inputs=3
  Mux1 : Mux  Inputs=3
  Mux2 : Mux  Inputs=3
  Out1 : Outport
  wires:
  In1/1 -> Demux/1
  Constant/1 -> Mux1/2, Mux/1, Mux2/3
  Demux/3 -> Mux/2, Gain1/1
  Demux/2 -> Gain/1, Mux2/1
  Gain/1 -> Mux/3
  Mux/1 -> Matrix Concatenation/1
  Gain1/1 -> Mux1/1
  Demux/1 -> Mux1/3, Gain2/1
  Mux1/1 -> Matrix Concatenation/2
  Mux2/1 -> Matrix Concatenation/3
  Gain2/1 -> Mux2/2
  Matrix Concatenation/1 -> Out1/1

== system collection_of_goodies/get pitch axis in ECI ==
  Q : Inport
  Math Function : Math  Operator=transpose
  Reshape : simulink/Math Operations/Reshape  OutputDimensionality=1-D array  OutputDimensions=[1,1]
  Selector : Selector  Elements=[4 5 6]  InputPortWidth=9
  pitch : Outport
  wires:
  Math Function/1 -> Reshape/1
  Reshape/1 -> Selector/1
  Q/1 -> Math Function/1
  Selector/1 -> pitch/1

== system collection_of_goodies/norm ==
  v : Inport
  Dot Product : simulink/Math Operations/Dot Product
  Math Function : Math  Operator=sqrt
  |v| : Outport
  wires:
  Math Function/1 -> |v|/1
  Dot Product/1 -> Math Function/1
  v/1 -> Dot Product/2, Dot Product/1

== system collection_of_goodies/normalize ==
  v : Inport
  Dot Product : simulink/Math Operations/Dot Product
  Math Function : Math  Operator=sqrt
  Product : Product  Inputs=*/  SaturateOnIntegerOverflow=on  InputSameDT=on
  v_hat : Outport
  wires:
  v/1 -> Dot Product/1, Dot Product/2, Product/1
  Dot Product/1 -> Math Function/1
  Math Function/1 -> Product/2
  Product/1 -> v_hat/1

== system collection_of_goodies/q1*inv(q2) ==
  q_B/N : Inport
  q_L/N : Inport  Port=2
  Mux : Mux  Inputs=2
  Mux1 : Mux
  qerr1 : Fcn  Expr=-u(4)*u(5)-u(3)*u(6)+u(2)*u(7)+u(1)*u(8)
  qerr2 : Fcn  Expr=u(3)*u(5)-u(4)*u(6)-u(1)*u(7)+u(2)*u(8)
  qerr3 : Fcn  Expr=-u(2)*u(5)+u(1)*u(6)-u(4)*u(7)+u(3)*u(8)
  qerr4 : Fcn  Expr=u(1)*u(5)+u(2)*u(6)+u(3)*u(7)+u(4)*u(8)
  q_B/L : Outport
  wires:
  q_B/N/1 -> Mux/1
  q_L/N/1 -> Mux/2
  Mux/1 -> qerr1/1, qerr2/1, qerr3/1, qerr4/1
  qerr1/1 -> Mux1/1
  qerr2/1 -> Mux1/2
  qerr3/1 -> Mux1/3
  qerr4/1 -> Mux1/4
  Mux1/1 -> q_B/L/1

== system collection_of_goodies/quat to DCM ==
  e0 e1 e2 e3 : Inport
  Demux : Demux
  Gain1 : Gain  Gain=2  SaturateOnIntegerOverflow=on
  Gain2 : Gain  Gain=2  SaturateOnIntegerOverflow=on
  Matrix Gain : Gain  Gain=eye(3,3)  SaturateOnIntegerOverflow=on
  Mux : Mux  Inputs=3
  Product : Product  SaturateOnIntegerOverflow=on  InputSameDT=on
  Product1 : Product  SaturateOnIntegerOverflow=on  InputSameDT=on
  Subsystem : Subsystem
      mask Display: disp('3x3 cross matrix')
  Sum1 : Sum  Inputs=|+-  SaturateOnIntegerOverflow=on  InputSameDT=on
  Sum8 : Sum  Inputs=|+-+  SaturateOnIntegerOverflow=on  InputSameDT=on
  T1 : Math  Operator=transpose
  T2 : Math  Operator=transpose
  qTq : Product  Multiplication=Matrix(*)  SaturateOnIntegerOverflow=on  InputSameDT=on
  qqT : Product  Multiplication=Matrix(*)  SaturateOnIntegerOverflow=on  InputSameDT=on
  DCM : Outport  InitialOutput=0
  wires:
  Sum8/1 -> DCM/1
  e0 e1 e2 e3/1 -> Demux/1
  Demux/1 -> Mux/1
  Demux/2 -> Mux/2
  Demux/3 -> Mux/3
  Demux/4 -> Product/2, Product1/1, Product1/2
  Mux/1 -> T1/1, qqT/1, Subsystem/1(In1), T2/1, qTq/2
  Product/1 -> Gain1/1
  T1/1 -> qqT/2
  qqT/1 -> Gain2/1
  Gain2/1 -> Sum8/1
  Gain1/1 -> Sum8/2
  Product1/1 -> Sum1/1
  T2/1 -> qTq/1
  qTq/1 -> Sum1/2
  Sum1/1 -> Matrix Gain/1
  Matrix Gain/1 -> Sum8/3
  Subsystem/1(Out1) -> Product/1

== system collection_of_goodies/quat_multiply (relative quat)1 ==
  q_bc : Inport
  q_ab : Inport  Port=2
  Mux : Mux  Inputs=2
  Mux1 : Mux
  qerr1 : Fcn  Expr=u(4)*u(5)+u(3)*u(6)-u(2)*u(7)+u(1)*u(8)
  qerr2 : Fcn  Expr=-u(3)*u(5)+u(4)*u(6)+u(1)*u(7)+u(2)*u(8)
  qerr3 : Fcn  Expr=u(2)*u(5)-u(1)*u(6)+u(4)*u(7)+u(3)*u(8)
  qerr4 : Fcn  Expr=-u(1)*u(5)-u(2)*u(6)-u(3)*u(7)+u(4)*u(8)
  q_ac : Outport
  wires:
  Mux1/1 -> q_ac/1
  qerr4/1 -> Mux1/4
  qerr3/1 -> Mux1/3
  qerr2/1 -> Mux1/2
  qerr1/1 -> Mux1/1
  Mux/1 -> qerr4/1, qerr3/1, qerr2/1, qerr1/1
  q_ab/1 -> Mux/2
  q_bc/1 -> Mux/1

== system collection_of_goodies/report difference from initial value ==
  In1 : Inport
  Constant : Constant
  Memory : Memory
  Memory1 : Memory
  Memory2 : Memory
  Sum : Sum  Inputs=|-+  SaturateOnIntegerOverflow=on
  Switch : Switch  Criteria=u2 > Threshold  Threshold=0.5  SaturateOnIntegerOverflow=on
  Out1 : Outport
  wires:
  Memory/1 -> Switch/2
  Constant/1 -> Memory/1
  In1/1 -> Switch/3, Memory2/1
  Switch/1 -> Memory1/1
  Memory1/1 -> Switch/1, Sum/1
  Sum/1 -> Out1/1
  Memory2/1 -> Sum/2

== system collection_of_goodies/rigid body ==
  External Torque : Inport
  Cross1 : Subsystem  Orientation=left
  Is : Gain  Orientation=left  Gain=Is  Multiplication=Matrix(K*u)  SaturateOnIntegerOverflow=on
  Is inverse : Gain  Gain=inv(Is)  Multiplication=Matrix(K*u)  SaturateOnIntegerOverflow=on
  Sum : Sum  Inputs=|+-  SaturateOnIntegerOverflow=on  InputSameDT=on
  "wbbn -> wbn" : Integrator  InitialCondition=wbn_init
  Angular rate : Outport
  wires:
  "wbbn -> wbn"/1 -> Cross1/1(A), Is/1, Angular rate/1
  Sum/1 -> Is inverse/1
  Is inverse/1 -> "wbbn -> wbn"/1
  Cross1/1(AxB) -> Sum/2
  Is/1 -> Cross1/2(B)
  External Torque/1 -> Sum/1

== system collection_of_goodies/row-wise  3x3-> 9x1 ==
  A(3x3) : Inport
  Demux7 : Demux  Outputs=9
  Mux4 : Mux  Inputs=9
  Reshape1 : simulink/Math Operations/Reshape  OutputDimensionality=Column vector  OutputDimensions=[1,1]
  A(9x1) : Outport
  wires:
  Reshape1/1 -> Demux7/1
  Demux7/9 -> Mux4/9
  Demux7/5 -> Mux4/5
  Demux7/1 -> Mux4/1
  Demux7/2 -> Mux4/4
  Demux7/3 -> Mux4/7
  Demux7/4 -> Mux4/2
  Demux7/6 -> Mux4/8
  Demux7/7 -> Mux4/3
  Demux7/8 -> Mux4/6
  Mux4/1 -> A(9x1)/1
  A(3x3)/1 -> Reshape1/1

== system collection_of_goodies/uncross ==
  v^x : Inport
  Demux : Demux  Outputs=9
  Mux : Mux  Inputs=3
  Reshape : simulink/Math Operations/Reshape  OutputDimensionality=1-D array  OutputDimensions=[1,1]
  Terminator{,1..5} (6 alike) : Terminator
  v : Outport
  wires:
  Mux/1 -> v/1
  v^x/1 -> Reshape/1
  Demux/1 -> Terminator/1
  Demux/5 -> Terminator1/1
  Demux/9 -> Terminator4/1
  Demux/8 -> Terminator5/1
  Demux/2 -> Mux/3
  Demux/4 -> Terminator2/1
  Demux/7 -> Mux/2
  Demux/3 -> Terminator3/1
  Demux/6 -> Mux/1
  Reshape/1 -> Demux/1

== system collection_of_goodies/AttError/qconjMult ==
  q_cmd : Inport
  q_est : Inport  Port=2
  Mux : Mux  Inputs=2
  Mux1 : Mux
  qerr1 : Fcn  Expr=-u(4)*u(5)-u(3)*u(6)+u(2)*u(7)+u(1)*u(8)
  qerr2 : Fcn  Expr=u(3)*u(5)-u(4)*u(6)-u(1)*u(7)+u(2)*u(8)
  qerr3 : Fcn  Expr=-u(2)*u(5)+u(1)*u(6)-u(4)*u(7)+u(3)*u(8)
  qerr4 : Fcn  Expr=u(1)*u(5)+u(2)*u(6)+u(3)*u(7)+u(4)*u(8)
  q_err : Outport
  wires:
  q_cmd/1 -> Mux/1
  q_est/1 -> Mux/2
  Mux/1 -> qerr1/1, qerr2/1, qerr3/1, qerr4/1
  qerr1/1 -> Mux1/1
  qerr2/1 -> Mux1/2
  qerr3/1 -> Mux1/3
  qerr4/1 -> Mux1/4
  Mux1/1 -> q_err/1

== system collection_of_goodies/AttitudeObserver/AttError ==
  q_meas : Inport  PortDimensions=4
  q_est : Inport  Port=2  PortDimensions=4
  Demux : Demux
  Gain : Gain  Gain=2  SaturateOnIntegerOverflow=on
  Mux : Mux  Inputs=3
  Terminator : Terminator
  qconjMult : Subsystem
  att_err : Outport
  wires:
  q_est/1 -> qconjMult/1(q_cmd)
  q_meas/1 -> qconjMult/2(q_est)
  qconjMult/1(q_err) -> Demux/1
  Demux/1 -> Mux/1
  Demux/2 -> Mux/2
  Demux/3 -> Mux/3
  Mux/1 -> Gain/1
  Gain/1 -> att_err/1
  Demux/4 -> Terminator/1

== system collection_of_goodies/AttitudeObserver/q_normalize ==
  q_in : Inport  PortDimensions=4
  Dot Product : simulink/Math Operations/Dot Product
  Math Function : Math  Operator=sqrt
  Product : Product  Inputs=*/  SaturateOnIntegerOverflow=on  InputSameDT=on
  q_out : Outport
  wires:
  q_in/1 -> Dot Product/1, Dot Product/2, Product/1
  Dot Product/1 -> Math Function/1
  Math Function/1 -> Product/2
  Product/1 -> q_out/1

== system collection_of_goodies/AttitudeObserver/qderiv ==
  w : Inport
  q : Inport  Port=2
  Mux : Mux  Inputs=2
  Mux1 : Mux
  qd1 : Fcn  Expr=(u(7)*u(1)-u(6)*u(2)+u(5)*u(3))/2
  qd2 : Fcn  Expr=(u(6)*u(1)+u(7)*u(2)-u(4)*u(3))/2
  qd3 : Fcn  Expr=(-u(5)*u(1)+u(4)*u(2)+u(7)*u(3))/2
  qd4 : Fcn  Expr=(-u(4)*u(1)-u(5)*u(2)-u(6)*u(3))/2
  qd : Outport
  wires:
  w/1 -> Mux/1
  q/1 -> Mux/2
  Mux/1 -> qd1/1, qd2/1, qd3/1, qd4/1
  qd1/1 -> Mux1/1
  qd2/1 -> Mux1/2
  qd3/1 -> Mux1/3
  qd4/1 -> Mux1/4
  Mux1/1 -> qd/1

== system collection_of_goodies/CMG Array Model/Array_Steering ==
  note: This Jacobian is NOT designed
      | to be singularity free
  gimbal_rate : Inport  PortDimensions=6
  spin_rate_meas : Inport  Port=2  PortDimensions=6
  gim_ang_meas : Inport  Port=3  PortDimensions=6
  Compute_Amatrix : Subsystem
  Cosine : Trigonometry  Operator=cos
  Dot Product : simulink/Math Operations/Dot Product
  Dot Product1 : simulink/Math Operations/Dot Product
  Dot Product2 : simulink/Math Operations/Dot Product
  Mux : Mux  Inputs=3
  Product : Product  SaturateOnIntegerOverflow=on  InputSameDT=on
  Product1 : Product  SaturateOnIntegerOverflow=on  InputSameDT=on
  Product2 : Product  SaturateOnIntegerOverflow=on  InputSameDT=on
  Sine : Trigonometry
  wheel_inertias : Constant  Value=wheel_inertias
  torque : Outport
  wires:
  Mux/1 -> torque/1
  Dot Product/1 -> Mux/1
  Dot Product2/1 -> Mux/3
  Dot Product1/1 -> Mux/2
  gimbal_rate/1 -> Dot Product2/2, Dot Product1/2, Dot Product/2
  Compute_Amatrix/3(Arow3) -> Dot Product2/1
  Compute_Amatrix/2(Arow2) -> Dot Product1/1
  Compute_Amatrix/1(Arow1) -> Dot Product/1
  Product2/1 -> Product1/1, Product/1
  wheel_inertias/1 -> Product2/1
  spin_rate_meas/1 -> Product2/2
  Cosine/1 -> Product1/2
  Sine/1 -> Product/2
  gim_ang_meas/1 -> Cosine/1, Sine/1
  Product1/1 -> Compute_Amatrix/2(cos_term)
  Product/1 -> Compute_Amatrix/1(sin_term)

== system collection_of_goodies/CMG Array Model/ComputeCMGMomentum ==
  spin_rate_meas : Inport  PortDimensions=6
  gim_ang_meas : Inport  Port=2  PortDimensions=6
  Cosine : Trigonometry  Operator=cos
  Product : Product  SaturateOnIntegerOverflow=on  InputSameDT=on
  Product1 : Product  SaturateOnIntegerOverflow=on  InputSameDT=on
  Product2 : Product  SaturateOnIntegerOverflow=on  InputSameDT=on
  Sine : Trigonometry
  Sum : Sum  SaturateOnIntegerOverflow=on  InputSameDT=on
  h_cos : Gain  Gain=h_cos_cmg  Multiplication=Matrix(K*u)  SaturateOnIntegerOverflow=on
  h_sin : Gain  Gain=h_sin_cmg  Multiplication=Matrix(K*u)  SaturateOnIntegerOverflow=on
  wheel_inertias : Constant  Value=wheel_inertias
  H_cmg : Outport
  wires:
  gim_ang_meas/1 -> Sine/1, Cosine/1
  Sine/1 -> Product/2
  Cosine/1 -> Product1/2
  h_sin/1 -> Sum/1
  h_cos/1 -> Sum/2
  spin_rate_meas/1 -> Product2/2
  wheel_inertias/1 -> Product2/1
  Product2/1 -> Product/1, Product1/1
  Sum/1 -> H_cmg/1
  Product1/1 -> h_cos/1
  Product/1 -> h_sin/1

== system collection_of_goodies/CMG Array Model/WxH (gyroscopic torque) ==
  v1 : Inport
  v2 : Inport  Port=2
  Cross1 : Fcn  Expr=-u(3)*u(5)+u(2)*u(6)
  Cross2 : Fcn  Expr=u(3)*u(4)-u(1)*u(6)
  Cross3 : Fcn  Expr=-u(2)*u(4)+u(1)*u(5)
  Mux : Mux  Inputs=2
  Mux1 : Mux  Inputs=3
  v1xv2 : Outport
  wires:
  v1/1 -> Mux/1
  v2/1 -> Mux/2
  Mux/1 -> Cross1/1, Cross2/1, Cross3/1
  Cross2/1 -> Mux1/2
  Cross1/1 -> Mux1/1
  Cross3/1 -> Mux1/3
  Mux1/1 -> v1xv2/1

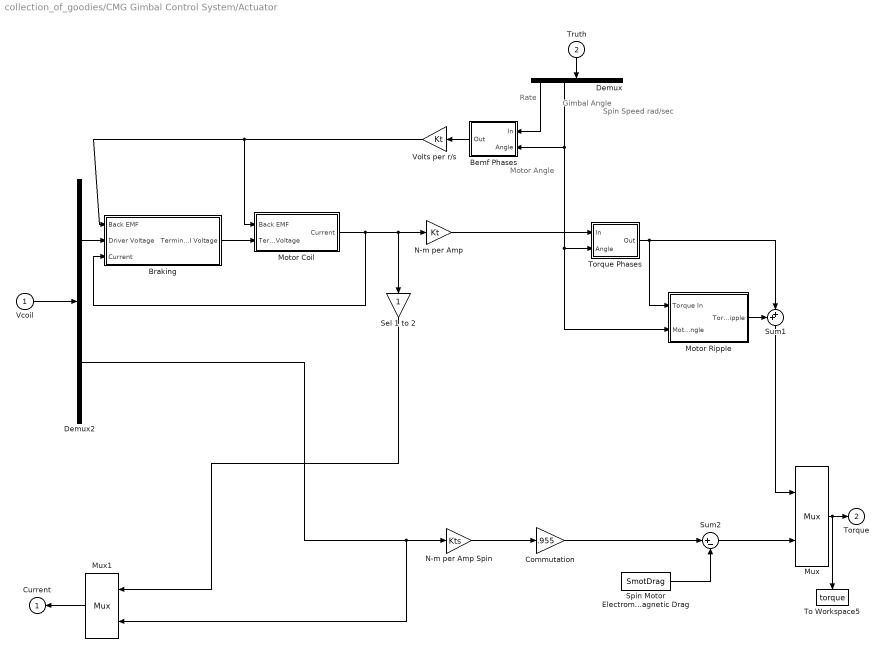
== system collection_of_goodies/CMG Gimbal Control System/Actuator ==
  note: Rate
  note: Motor Angle
  note: Spin
      | Speed
      | rad/sec
  note: Gimbal
      | Angle
  Vcoil : Inport
  Truth : Inport  Orientation=down  Port=2
  Bemf Phases : Subsystem  Orientation=left
  Braking : Subsystem
  Commutation : Gain  Gain=.955  SaturateOnIntegerOverflow=on
  Demux : Demux  Orientation=down
  Demux2 : Demux  Outputs=[2 1]
  Motor Coil : Subsystem
  Motor Ripple : Subsystem
  Mux : Mux  Inputs=2
  Mux1 : Mux  Orientation=left  Inputs=[2 1]
  N-m per Amp : Gain  Gain=Kt  SaturateOnIntegerOverflow=on
  N-m per Amp Spin : Gain  Gain=Kts  SaturateOnIntegerOverflow=on
  Sel 1 to 2 : Gain  Orientation=down  SaturateOnIntegerOverflow=on
  Spin Motor Electromagnetic Drag : Constant  Value=SmotDrag
  Sum1 : Sum  Orientation=down  Inputs=++|  SaturateOnIntegerOverflow=on  InputSameDT=on
  Sum2 : Sum  Inputs=|+-  SaturateOnIntegerOverflow=on  InputSameDT=on
  To Workspace5 : ToWorkspace  VariableName=torque  SampleTime=-1  SaveFormat=Array
      settings: Orientation=down
  Torque Phases : Subsystem
  Volts per r/s : Gain  Orientation=left  Gain=Kt  SaturateOnIntegerOverflow=on
  Current : Outport  Orientation=left  InitialOutput=0
  Torque : Outport  Port=2  InitialOutput=0
  wires:
  Mux1/1 -> Current/1
  Bemf Phases/1(Out) -> Volts per r/s/1
  N-m per Amp/1 -> Torque Phases/1(In)
  Sel 1 to 2/1 -> Mux1/1
  Spin Motor Electromagnetic Drag/1 -> Sum2/2
  Sum2/1 -> Mux/2
  Mux/1 -> Torque/1, To Workspace5/1
  Demux/1 -> Bemf Phases/1(In)
  Motor Ripple/1(Torque Ripple) -> Sum1/1
  Sum1/1 -> Mux/1
  Truth/1 -> Demux/1
  Demux/2 -> Bemf Phases/2(Angle), Torque Phases/2(Angle), Motor Ripple/2(Motor Angle)
  Torque Phases/1(Out) -> Motor Ripple/1(Torque In), Sum1/2
  N-m per Amp Spin/1 -> Commutation/1
  Commutation/1 -> Sum2/1
  Braking/1(Terminal Voltage) -> Motor Coil/2(Terminal Voltage)
  Motor Coil/1(Current) -> N-m per Amp/1, Sel 1 to 2/1, Braking/3(Current)
  Volts per r/s/1 -> Motor Coil/1(Back EMF), Braking/1(Back EMF)
  Demux2/2 -> N-m per Amp Spin/1, Mux1/2
  Demux2/1 -> Braking/2(Driver Voltage)
  Vcoil/1 -> Demux2/1

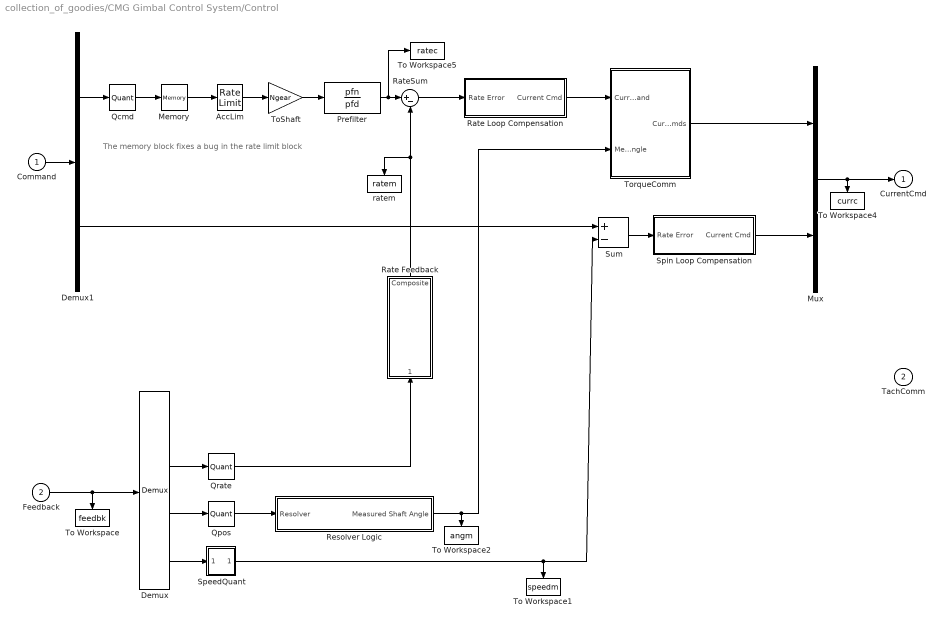
== system collection_of_goodies/CMG Gimbal Control System/Control ==
  note: The memory block fixes
      | a bug in the rate limit block
  Command : Inport  PortDimensions=2
  Feedback : Inport  Port=2
  AccLim : RateLimiter  RisingSlewLimit=AccLim  FallingSlewLimit=-AccLim
  Demux : Demux  Outputs=[3 2 4 1]
  Demux1 : Demux  Outputs=2
  Memory : Memory
  Mux : Mux  Inputs=[2 1]
  Prefilter : TransferFcn  Numerator=pfn  Denominator=pfd
  Qcmd : Quantizer  QuantizationInterval=Qcmd
  Qpos : Quantizer  QuantizationInterval=Qpos
  Qrate : Quantizer  QuantizationInterval=Qrate
  Rate Feedback : Subsystem  Orientation=up
  Rate Loop Compensation : Subsystem
  RateSum : Sum  Inputs=|+-  SaturateOnIntegerOverflow=on  InputSameDT=on
  Resolver Logic : Subsystem
  SpeedQuant : Subsystem
  Spin Loop Compensation : Subsystem
  Sum : Sum  Inputs=+-  SaturateOnIntegerOverflow=on  InputSameDT=on
  To Workspace : ToWorkspace  VariableName=feedbk  SampleTime=-1  SaveFormat=Array
      settings: Orientation=down
  To Workspace1 : ToWorkspace  VariableName=speedm  SampleTime=-1  SaveFormat=Array
      settings: Orientation=down
  To Workspace2 : ToWorkspace  VariableName=angm  SampleTime=-1  SaveFormat=Array
      settings: Orientation=down
  To Workspace4 : ToWorkspace  VariableName=currc  SampleTime=-1  SaveFormat=Array
      settings: Orientation=down
  To Workspace5 : ToWorkspace  VariableName=ratec  SampleTime=-1  SaveFormat=Array
  ToShaft : Gain  Gain=Ngear
  TorqueComm : Subsystem
  ratem : ToWorkspace  VariableName=ratem  SampleTime=-1  SaveFormat=Array
      settings: Orientation=down
  CurrentCmd : Outport  InitialOutput=0
  TachComm : Outport  Port=2  InitialOutput=0
  wires:
  Demux/2 -> Qrate/1
  Demux/3 -> Qpos/1
  Qpos/1 -> Resolver Logic/1(Resolver)
  Demux/4 -> SpeedQuant/1(In)
  SpeedQuant/1(Out) -> Sum/2, To Workspace1/1
  Resolver Logic/1(Measured Shaft Angle) -> TorqueComm/2(Meas Shaft Angle), To Workspace2/1
  Feedback/1 -> Demux/1, To Workspace/1
  Command/1 -> Demux1/1
  Qrate/1 -> Rate Feedback/1(Coarse/Fine)
  Qcmd/1 -> Memory/1
  AccLim/1 -> ToShaft/1
  Demux1/1 -> Qcmd/1
  Memory/1 -> AccLim/1
  TorqueComm/1(Current Cmds) -> Mux/1
  ToShaft/1 -> Prefilter/1
  Prefilter/1 -> RateSum/1, To Workspace5/1
  Sum/1 -> Spin Loop Compensation/1(Rate Error)
  Spin Loop Compensation/1(Current Cmd) -> Mux/2
  Demux1/2 -> Sum/1
  Mux/1 -> CurrentCmd/1, To Workspace4/1
  Rate Feedback/1(Composite) -> RateSum/2, ratem/1
  RateSum/1 -> Rate Loop Compensation/1(Rate Error)
  Rate Loop Compensation/1(Current Cmd) -> TorqueComm/1(Current Command)

== system collection_of_goodies/CMG Gimbal Control System/Drive ==
  Current : Inport
  CurrentCmd : Inport  Port=2
  Current Loop 1 : Subsystem
  Current Loop 2 : Subsystem
  Demux1 : Demux  Outputs=3
  Demux2 : Demux  Outputs=3
  Mux : Mux  Inputs=3
  Mux1 : Mux  Inputs=3
  To Workspace4 : ToWorkspace  VariableName=curr  SampleTime=-1  SaveFormat=Array
      settings: Orientation=down
  To Workspace5 : ToWorkspace  VariableName=vcoil  SampleTime=-1  SaveFormat=Array
      settings: Orientation=down
  Vcoil : Outport  InitialOutput=0
  CurSense : Outport  Port=2  InitialOutput=0
  wires:
  CurrentCmd/1 -> Demux1/1
  Demux1/3 -> Mux/3
  Mux1/1 -> CurSense/1
  Demux2/3 -> Mux1/3
  Demux1/1 -> Current Loop 1/1(CurrentCmd)
  Demux1/2 -> Current Loop 2/1(CurrentCmd)
  Demux2/1 -> Current Loop 1/2(Current)
  Demux2/2 -> Current Loop 2/2(Current)
  Current Loop 1/1(Vanalog) -> Mux/1
  Current Loop 2/1(Vanalog) -> Mux/2
  Current Loop 1/2(CurSense) -> Mux1/1
  Current Loop 2/2(CurSense) -> Mux1/2
  Current/1 -> Demux2/1, To Workspace4/1
  Mux/1 -> Vcoil/1, To Workspace5/1

== system collection_of_goodies/CMG Gimbal Control System/Sensor ==
  note: Motor Angle
  note: Gimbal Angle
  note: Motor
      | Rate
  TachComm : Inport
  CurSense : Inport  Port=2
  Truth : Inport  Port=3
  AAF : TransferFcn  Denominator=TachAAFd
  Demux : Demux
  Fine Gain : Gain  Gain=fine  SaturateOnIntegerOverflow=on
  Mux : Mux  Inputs=[3 1 1 4 1]
  Resolvers : Subsystem
  Tach Phases : Subsystem
  Tach Ripple : Subsystem
  Tachometer : Sum  Inputs=|++  SaturateOnIntegerOverflow=on  InputSameDT=on
  Sensor : Outport  InitialOutput=0
  wires:
  Mux/1 -> Sensor/1
  Tach Phases/1(Meas Rate) -> AAF/1
  Fine Gain/1 -> Mux/3
  Tachometer/1 -> Tach Phases/2(Rate)
  CurSense/1 -> Mux/1
  TachComm/1 -> Tach Phases/1(TachComm)
  AAF/1 -> Mux/2, Fine Gain/1
  Demux/2 -> Tach Ripple/2(Motor Angle), Tach Phases/3(Truth Angle), Resolvers/1(Truth Angle)
  Resolvers/1(Resolver Out) -> Mux/4
  Demux/1 -> Tachometer/1, Tach Ripple/1(Rate In)
  Tach Ripple/1(Tach Ripple) -> Tachometer/2
  Truth/1 -> Demux/1
  Demux/4 -> Mux/5
